simulink model "Process_test"  (Simulink 7.9)
settings: Solver=ode45  StartTime=0.0  StopTime=10.0  RelTol=1e-3
values from neighbouring files (symbols this model uses):
  h = Ts_kalman    (= 0.01)    [MPC_setup_nonlinear.m]    (also in real_phi_ref.mat; real_phi_ref_2.mat; real_phi_ref_temp.mat; real_theta_constraint.mat)
settings Model: Creator=tna13skn  LastModifiedBy=tna13skn

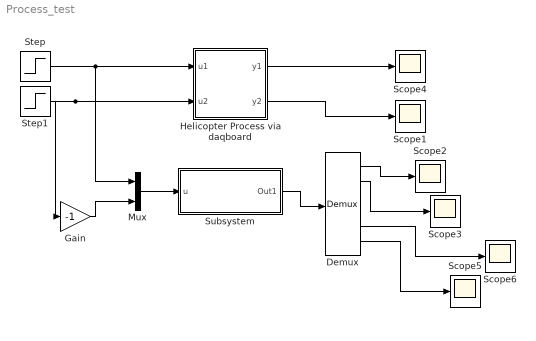
== system Process_test ==
  Demux : Demux  Outputs=6
  Gain : Gain  Gain=-1
  Helicopter Process via daqboard : Subsystem
  Mux : Mux  Inputs=2
  Scope{1..6} (6 alike) : Scope
      Scope1 settings: SaveName=ScopeData2
      Scope2 settings: YMin=0  YMax=15  SaveName=ScopeData3
      Scope3 settings: SaveName=ScopeData4
      Scope5 settings: SaveName=ScopeData5
      Scope6 settings: SaveName=ScopeData6
  Step : Step  After=0  SampleTime=0
  Step1 : Step  After=0  SampleTime=0  ZeroCross=off
  Subsystem : Subsystem
  wires:
  Step/1 -> Helicopter Process via daqboard/1(u1), Mux/1
  Step1/1 -> Helicopter Process via daqboard/2(u2), Gain/1
  Helicopter Process via daqboard/1(y1) -> Scope4/1
  Helicopter Process via daqboard/2(y2) -> Scope1/1
  Mux/1 -> Subsystem/1(u)
  Subsystem/1(Out1) -> Demux/1
  Demux/1 -> Scope2/1
  Demux/2 -> Scope3/1
  Demux/6 -> Scope5/1
  Demux/5 -> Scope6/1
  Gain/1 -> Mux/2

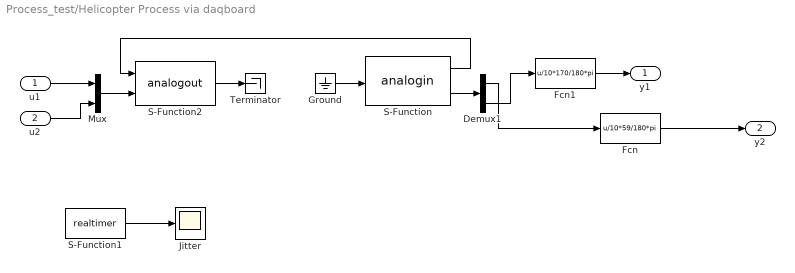
== system Process_test/Helicopter Process via daqboard ==
  u1 : Inport
  u2 : Inport  Port=2
  Demux1 : Demux  Outputs=2
  Fcn : Fcn  Expr=u/10*59/180*pi
  Fcn1 : Fcn  Expr=u/10*170/180*pi
  Ground : Ground
  Jitter : Scope
  Mux : Mux  Inputs=2
  S-Function : S-Function  FunctionName=analogin  Parameters=h [0 1]  EnableBusSupport=off
  S-Function1 : S-Function  FunctionName=realtimer  Parameters=h  EnableBusSupport=off
  S-Function2 : S-Function  FunctionName=analogout  Parameters=h [0 1]  EnableBusSupport=off
  Terminator : Terminator
  y1 : Outport  InitialOutput=0
  y2 : Outport  Port=2  InitialOutput=0
  wires:
  S-Function1/1 -> Jitter/1
  Mux/1 -> S-Function2/2
  Demux1/2 -> Fcn1/1
  Demux1/1 -> Fcn/1
  S-Function/2 -> Demux1/1
  u2/1 -> Mux/2
  u1/1 -> Mux/1
  Ground/1 -> S-Function/1
  S-Function2/1 -> Terminator/1
  S-Function/1 -> S-Function2/1
  Fcn/1 -> y2/1
  Fcn1/1 -> y1/1

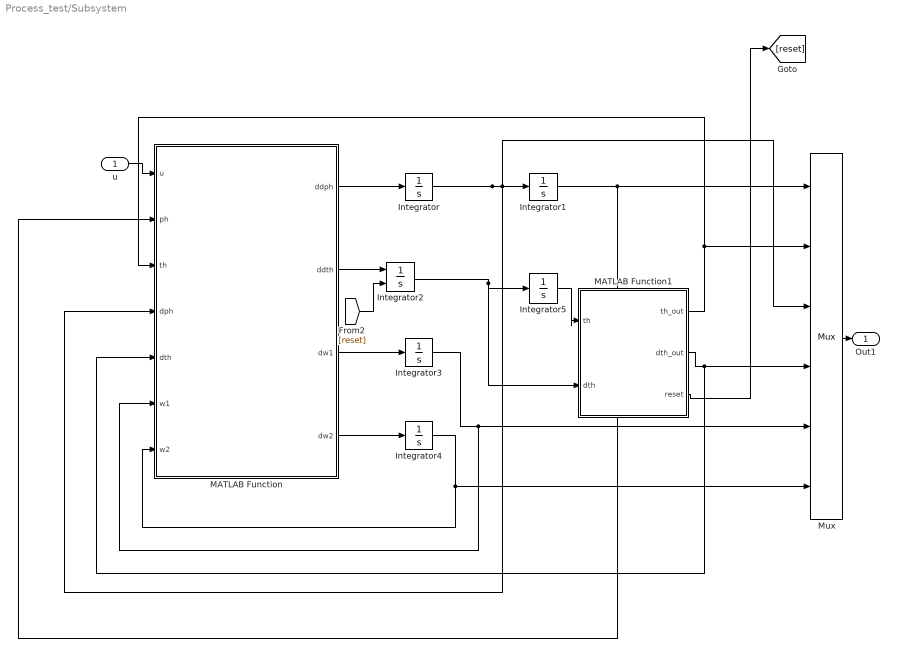
== system Process_test/Subsystem ==
  u : Inport
  Integrator{,1,3..4} (4 alike) : Integrator
  Integrator2 : Integrator  ExternalReset=rising  ShowStatePort=on
  Integrator5 : Integrator  ShowStatePort=on
  MATLAB Function : MATLAB Function  TreatAsAtomicUnit=on
  MATLAB Function1 : MATLAB Function  TreatAsAtomicUnit=on
  Mux : Mux  Inputs=6
  Out1 : Outport
  wires:
  u/1 -> MATLAB Function/1(u)
  MATLAB Function/1(ddph) -> Integrator/1
  Integrator/1 -> Integrator1/1, MATLAB Function/4(dph), Mux/3
  Integrator1/1 -> Mux/1, MATLAB Function/2(ph)
  Mux/1 -> Out1/1
  MATLAB Function/2(ddth) -> Integrator2/1
  MATLAB Function/3(dw1) -> Integrator3/1
  MATLAB Function/4(dw2) -> Integrator4/1
  Integrator4/1 -> Mux/6, MATLAB Function/7(w2)
  Integrator3/1 -> Mux/5, MATLAB Function/6(w1)
  [reset] -> Integrator2/2
  MATLAB Function1/1(th_out) -> Mux/2, MATLAB Function/3(th)
  MATLAB Function1/2(dth_out) -> Mux/4, MATLAB Function/5(dth)
  Integrator5/1 -> MATLAB Function1/1(th)
  Integrator2/1 -> MATLAB Function1/2(dth), Integrator5/1
  MATLAB Function1/3(reset) -> [reset]

== matlab function Subsystem/MATLAB Function ==
  data: u input double; ddph output double; ph input double; th input double; dph input double; dth input double; w1 input double; w2 input double; ddth output double; dw1 output double; dw2 output double
function [ddph, ddth, dw1, dw2] = fcn(u, ph, th, dph, dth, w1, w2)
% Implementation of the non-linear integration model derived in the
% technical report "Modelling of the ETH Helicopter Laboratory Process"
% by Magnus Gäfvert, implemented by Marcus Greiff for the project course in
% FRTN01/FRTN15 2018-03-18. The notation and nomenclature vollows the
% report, however, the state vector is defined as
%
%   $x \triangleq [phi; theta; \dot{phi}; \dot{theta}; \omega_1; \omega_2]$
%
% The parameters in Gäfverts report are hard coded in the non-linear model,
% but will be made more general in future revisions.


%% Parameters
% Weights
ml = 0.280;  % [kg]
m1 = 0.3792; % [kg]
m2 = 0.1739; % [kg]
mw = 0.158;  % [kg]
m  = ml + m1 + m2 + mw; % [kg] (eq. 24)

% Distances
l1 = 0.1995; % [m]
l2 = 0.1743; % [m]
lw = 0.090;  % [m]
h  = 0.0298; % [m]
lc = (ml*(l1-l2)+m1*l1-m2*l2-mw*lw)/m; % [m] (eq. 27)

% Inertial parameters
g = 9.81; % [m/s^2]
Ja = 0;   % [] (eq. 26)
Jl = (ml/3)*((l1^3+l2^3)/(l1+l2))+m1*l1^2+m2*l2^2+mw*lw^2; % [] (eq. 25)

% Time, motor and aerodynamics constants
k1 = 1.00e-2; % [Vs/rad]
k2 = 1.39e-2; % [Vs/rad]
C1 = 2.50e-5; % [Ns^/rad^2]
C2 = 1.58e-6; % [Ns^/rad^2]
D1 = 2.90e-7; % [Nms^/rad^2]
D2 = 1.76e-7; % [Nms^/rad^2]
T1 = 1.10;    % [s]
T2 = 0.33;    % [s]


%% Pre-computation of angles and extraction of states
cth = cos(th);
sth = sin(th);
u1 = u(1);
u2 = u(2);

%%rotation stop


%% Integration model
ddph = (cth^2*Jl - 2*h*cth*sth*m*lc + h^2*sth^2*m + Ja)\...
       (2*cth*sth*dph*dth*Jl - 2*h*(sth^2-cth^2)*dph*dth*m*lc - ...
	2*h^2*sth*cth*dph*dth*m + D1*w1*abs(w1)*cth + l2*cth*C2*w2*abs(w2));
ddth = (Jl + h^2*m)\...
       (-cth*sth*dph^2*Jl - h*(-sth^2+cth^2)*dph^2*m*lc - g*cth*m*lc ...
	+ h^2*sth*cth*dph^2*m + m*g*h*sth + l1*C1*w1*abs(w1) + D2*w2*abs(w2));
dw1 = -w1/T1 + u1/(k1*T1);
dw2 = -w2/T2 + u2/(k2*T2);

if(th<=-pi/4&&dth<=0&&ddth<0)
    ddth=0;
end

== matlab function Subsystem/MATLAB Function1 ==
  data: th input double; th_out output double; dth input double; dth_out output double; reset output double
function [th_out,dth_out,reset] = fcn(th,dth)

if(th<=-pi/4&&dth<0)
    th_out=-pi/4;
    dth_out=0;
    reset=1;
    
else
    th_out=th;
    dth_out=dth; 
    reset=0;
end
